simulink model "sensors_actuators"  (Simulink 6.4)
settings: Solver=ode45  StartTime=0.0  StopTime=10.0  RelTol=1e-3
undefined symbols (not defined in the file or in its folder): max_XXX, min_XXX, noiseseed_XXX, noisesource_XXX, std_XXX, T0_XXX, T_XXX, useideal_XXX, usenoise_XXX, XXX
settings Model: Creator=ielulf  LastModifiedBy=ielulf  ExtModeAutoUpdateStatusClock=off

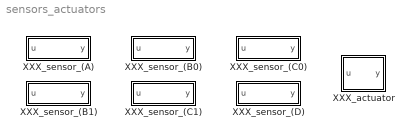
== system sensors_actuators ==
  XXX_actuator : Subsystem
  XXX_sensor_(A) : Subsystem
  XXX_sensor_(B0) : Subsystem
  XXX_sensor_(B1) : Subsystem
  XXX_sensor_(C0) : Subsystem
  XXX_sensor_(C1) : Subsystem
  XXX_sensor_(D) : Subsystem

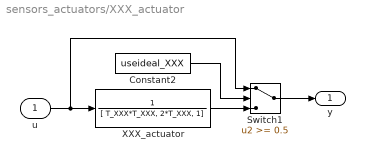
== system sensors_actuators/XXX_actuator ==
  u : Inport
  Constant2 : Constant  Value=useideal_XXX
  Switch1 : Switch  Threshold=0.5
  XXX_actuator : TransferFcn  Denominator=[ T_XXX*T_XXX, 2*T_XXX, 1]
  y : Outport
  wires:
  Constant2/1 -> Switch1/2
  XXX_actuator/1 -> Switch1/3
  Switch1/1 -> y/1
  u/1 -> Switch1/1, XXX_actuator/1

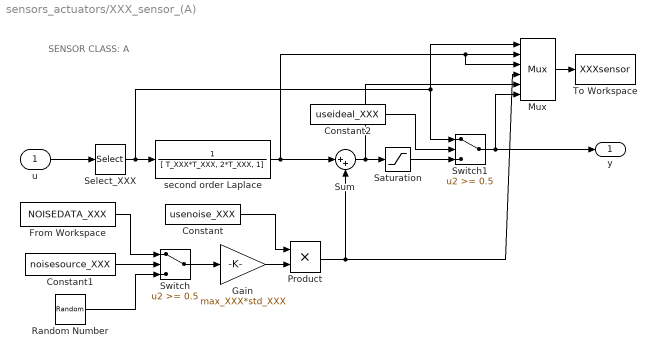
== system sensors_actuators/XXX_sensor_(A) ==
  note: SENSOR CLASS: A
  u : Inport
  Constant : Constant  Value=usenoise_XXX
  Constant1 : Constant  Value=noisesource_XXX
  Constant2 : Constant  Value=useideal_XXX
  From Workspace : FromWorkspace  VariableName=NOISEDATA_XXX  SampleTime=0
  Gain : Gain  Gain=max_XXX*std_XXX  SaturateOnIntegerOverflow=on
  Mux : Mux  Inputs=6
  Product : Product  SaturateOnIntegerOverflow=on  InputSameDT=on
  Random Number : RandomNumber  Seed=noiseseed_XXX  SampleTime=1/1440
  Saturation : Saturate  UpperLimit=max_XXX  LowerLimit=min_XXX
  Select_XXX : Selector  Elements=[XXX]  InputPortWidth=15
  Sum : Sum  Inputs=|++  SaturateOnIntegerOverflow=on  InputSameDT=on
  Switch : Switch  Threshold=0.5
  Switch1 : Switch  Threshold=0.5
  To Workspace : ToWorkspace  VariableName=XXXsensor  SampleTime=-1  SaveFormat=Array
  second order Laplace : TransferFcn  Denominator=[ T_XXX*T_XXX, 2*T_XXX, 1]
  y : Outport
  wires:
  Sum/1 -> Saturation/1, Mux/5
  second order Laplace/1 -> Sum/1, Mux/2, Mux/3
  Product/1 -> Sum/2, Mux/4
  u/1 -> Select_XXX/1
  Select_XXX/1 -> second order Laplace/1, Switch1/1, Mux/1
  Gain/1 -> Product/2
  Switch/1 -> Gain/1
  Constant/1 -> Product/1
  From Workspace/1 -> Switch/1
  Constant1/1 -> Switch/2
  Random Number/1 -> Switch/3
  Saturation/1 -> Switch1/3
  Switch1/1 -> y/1, Mux/6
  Constant2/1 -> Switch1/2
  Mux/1 -> To Workspace/1

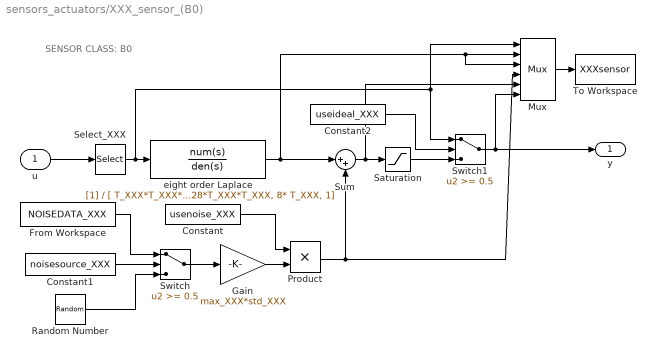
== system sensors_actuators/XXX_sensor_(B0) ==
  note: SENSOR CLASS: B0
  u : Inport
  Constant : Constant  Value=usenoise_XXX
  Constant1 : Constant  Value=noisesource_XXX
  Constant2 : Constant  Value=useideal_XXX
  From Workspace : FromWorkspace  VariableName=NOISEDATA_XXX  SampleTime=0
  Gain : Gain  Gain=max_XXX*std_XXX  SaturateOnIntegerOverflow=on
  Mux : Mux  Inputs=6
  Product : Product  SaturateOnIntegerOverflow=on  InputSameDT=on
  Random Number : RandomNumber  Seed=noiseseed_XXX  SampleTime=1/1440
  Saturation : Saturate  UpperLimit=max_XXX  LowerLimit=min_XXX
  Select_XXX : Selector  Elements=[XXX]  InputPortWidth=15
  Sum : Sum  Inputs=|++  SaturateOnIntegerOverflow=on  InputSameDT=on
  Switch : Switch  Threshold=0.5
  Switch1 : Switch  Threshold=0.5
  To Workspace : ToWorkspace  VariableName=XXXsensor  SampleTime=-1  SaveFormat=Array
  eight order Laplace : TransferFcn  Denominator=[ T_XXX*T_XXX*T_XXX*T_XXX*T_XXX*T_XXX*T_XXX*T_XXX, 8*T_XXX*T_XXX*T_XXX*T_XXX*T_XXX*T_XXX*T_XXX, 28*T_XXX*T_XXX*T_XXX*T_XXX*T_XXX*T_XXX, 56*T_XXX*T_XXX*T_XXX*T_XXX*T_XXX, 70*T_XXX*T_XXX*T_XXX*T_XXX, 56*T_XXX*T_XXX*T_XXX, 28*T_XXX*T_XXX, 8* T_XXX, 1]
  y : Outport
  wires:
  Sum/1 -> Saturation/1, Mux/5
  eight order Laplace/1 -> Sum/1, Mux/2, Mux/3
  Product/1 -> Sum/2, Mux/4
  u/1 -> Select_XXX/1
  Select_XXX/1 -> eight order Laplace/1, Switch1/1, Mux/1
  Gain/1 -> Product/2
  Switch/1 -> Gain/1
  Constant/1 -> Product/1
  From Workspace/1 -> Switch/1
  Constant1/1 -> Switch/2
  Random Number/1 -> Switch/3
  Saturation/1 -> Switch1/3
  Switch1/1 -> y/1, Mux/6
  Constant2/1 -> Switch1/2
  Mux/1 -> To Workspace/1

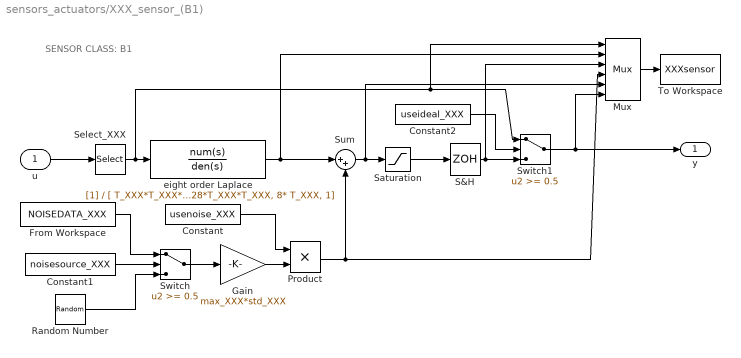
== system sensors_actuators/XXX_sensor_(B1) ==
  note: SENSOR CLASS: B1
  u : Inport
  Constant : Constant  Value=usenoise_XXX
  Constant1 : Constant  Value=noisesource_XXX
  Constant2 : Constant  Value=useideal_XXX
  From Workspace : FromWorkspace  VariableName=NOISEDATA_XXX  SampleTime=0
  Gain : Gain  Gain=max_XXX*std_XXX  SaturateOnIntegerOverflow=on
  Mux : Mux  Inputs=6
  Product : Product  SaturateOnIntegerOverflow=on  InputSameDT=on
  Random Number : RandomNumber  Seed=noiseseed_XXX  SampleTime=1/1440
  S&H : ZeroOrderHold  SampleTime=T0_XXX
  Saturation : Saturate  UpperLimit=max_XXX  LowerLimit=min_XXX
  Select_XXX : Selector  Elements=[XXX]  InputPortWidth=15
  Sum : Sum  Inputs=|++  SaturateOnIntegerOverflow=on  InputSameDT=on
  Switch : Switch  Threshold=0.5
  Switch1 : Switch  Threshold=0.5
  To Workspace : ToWorkspace  VariableName=XXXsensor  SampleTime=-1  SaveFormat=Array
  eight order Laplace : TransferFcn  Denominator=[ T_XXX*T_XXX*T_XXX*T_XXX*T_XXX*T_XXX*T_XXX*T_XXX, 8*T_XXX*T_XXX*T_XXX*T_XXX*T_XXX*T_XXX*T_XXX, 28*T_XXX*T_XXX*T_XXX*T_XXX*T_XXX*T_XXX, 56*T_XXX*T_XXX*T_XXX*T_XXX*T_XXX, 70*T_XXX*T_XXX*T_XXX*T_XXX, 56*T_XXX*T_XXX*T_XXX, 28*T_XXX*T_XXX, 8* T_XXX, 1]
  y : Outport
  wires:
  Switch1/1 -> Mux/6, y/1
  Constant2/1 -> Switch1/2
  S&H/1 -> Mux/3, Switch1/3
  Saturation/1 -> S&H/1
  Sum/1 -> Saturation/1, Mux/5
  eight order Laplace/1 -> Mux/2, Sum/1
  Product/1 -> Sum/2, Mux/4
  u/1 -> Select_XXX/1
  Select_XXX/1 -> Switch1/1, Mux/1, eight order Laplace/1
  Gain/1 -> Product/2
  Switch/1 -> Gain/1
  Constant/1 -> Product/1
  From Workspace/1 -> Switch/1
  Constant1/1 -> Switch/2
  Random Number/1 -> Switch/3
  Mux/1 -> To Workspace/1

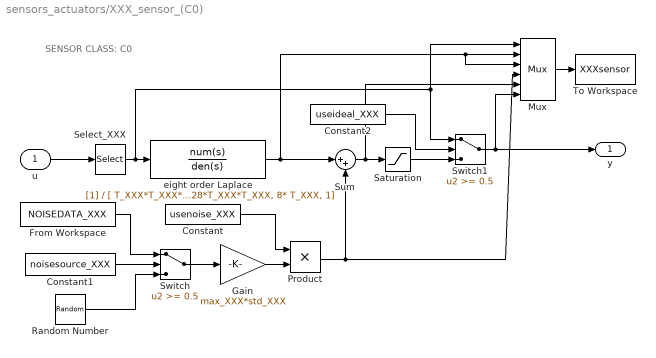
== system sensors_actuators/XXX_sensor_(C0) ==
  note: SENSOR CLASS: C0
  u : Inport
  Constant : Constant  Value=usenoise_XXX
  Constant1 : Constant  Value=noisesource_XXX
  Constant2 : Constant  Value=useideal_XXX
  From Workspace : FromWorkspace  VariableName=NOISEDATA_XXX  SampleTime=0
  Gain : Gain  Gain=max_XXX*std_XXX  SaturateOnIntegerOverflow=on
  Mux : Mux  Inputs=6
  Product : Product  SaturateOnIntegerOverflow=on  InputSameDT=on
  Random Number : RandomNumber  Seed=noiseseed_XXX  SampleTime=1/1440
  Saturation : Saturate  UpperLimit=max_XXX  LowerLimit=min_XXX
  Select_XXX : Selector  Elements=[XXX]  InputPortWidth=15
  Sum : Sum  Inputs=|++  SaturateOnIntegerOverflow=on  InputSameDT=on
  Switch : Switch  Threshold=0.5
  Switch1 : Switch  Threshold=0.5
  To Workspace : ToWorkspace  VariableName=XXXsensor  SampleTime=-1  SaveFormat=Array
  eight order Laplace : TransferFcn  Denominator=[ T_XXX*T_XXX*T_XXX*T_XXX*T_XXX*T_XXX*T_XXX*T_XXX, 8*T_XXX*T_XXX*T_XXX*T_XXX*T_XXX*T_XXX*T_XXX, 28*T_XXX*T_XXX*T_XXX*T_XXX*T_XXX*T_XXX, 56*T_XXX*T_XXX*T_XXX*T_XXX*T_XXX, 70*T_XXX*T_XXX*T_XXX*T_XXX, 56*T_XXX*T_XXX*T_XXX, 28*T_XXX*T_XXX, 8* T_XXX, 1]
  y : Outport
  wires:
  Sum/1 -> Saturation/1, Mux/5
  eight order Laplace/1 -> Sum/1, Mux/2, Mux/3
  Product/1 -> Sum/2, Mux/4
  u/1 -> Select_XXX/1
  Select_XXX/1 -> eight order Laplace/1, Switch1/1, Mux/1
  Gain/1 -> Product/2
  Switch/1 -> Gain/1
  Constant/1 -> Product/1
  From Workspace/1 -> Switch/1
  Constant1/1 -> Switch/2
  Random Number/1 -> Switch/3
  Saturation/1 -> Switch1/3
  Switch1/1 -> y/1, Mux/6
  Constant2/1 -> Switch1/2
  Mux/1 -> To Workspace/1

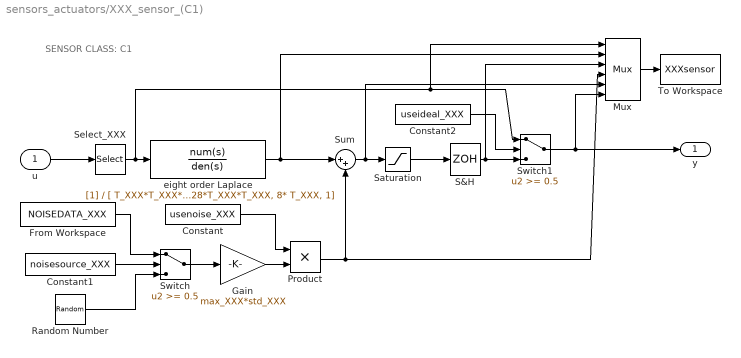
== system sensors_actuators/XXX_sensor_(C1) ==
  note: SENSOR CLASS: C1
  u : Inport
  Constant : Constant  Value=usenoise_XXX
  Constant1 : Constant  Value=noisesource_XXX
  Constant2 : Constant  Value=useideal_XXX
  From Workspace : FromWorkspace  VariableName=NOISEDATA_XXX  SampleTime=0
  Gain : Gain  Gain=max_XXX*std_XXX  SaturateOnIntegerOverflow=on
  Mux : Mux  Inputs=6
  Product : Product  SaturateOnIntegerOverflow=on  InputSameDT=on
  Random Number : RandomNumber  Seed=noiseseed_XXX  SampleTime=1/1440
  S&H : ZeroOrderHold  SampleTime=T0_XXX
  Saturation : Saturate  UpperLimit=max_XXX  LowerLimit=min_XXX
  Select_XXX : Selector  Elements=[XXX]  InputPortWidth=15
  Sum : Sum  Inputs=|++  SaturateOnIntegerOverflow=on  InputSameDT=on
  Switch : Switch  Threshold=0.5
  Switch1 : Switch  Threshold=0.5
  To Workspace : ToWorkspace  VariableName=XXXsensor  SampleTime=-1  SaveFormat=Array
  eight order Laplace : TransferFcn  Denominator=[ T_XXX*T_XXX*T_XXX*T_XXX*T_XXX*T_XXX*T_XXX*T_XXX, 8*T_XXX*T_XXX*T_XXX*T_XXX*T_XXX*T_XXX*T_XXX, 28*T_XXX*T_XXX*T_XXX*T_XXX*T_XXX*T_XXX, 56*T_XXX*T_XXX*T_XXX*T_XXX*T_XXX, 70*T_XXX*T_XXX*T_XXX*T_XXX, 56*T_XXX*T_XXX*T_XXX, 28*T_XXX*T_XXX, 8* T_XXX, 1]
  y : Outport
  wires:
  Switch1/1 -> Mux/6, y/1
  Constant2/1 -> Switch1/2
  S&H/1 -> Mux/3, Switch1/3
  Saturation/1 -> S&H/1
  Sum/1 -> Saturation/1, Mux/5
  eight order Laplace/1 -> Mux/2, Sum/1
  Product/1 -> Sum/2, Mux/4
  u/1 -> Select_XXX/1
  Select_XXX/1 -> Switch1/1, Mux/1, eight order Laplace/1
  Gain/1 -> Product/2
  Switch/1 -> Gain/1
  Constant/1 -> Product/1
  From Workspace/1 -> Switch/1
  Constant1/1 -> Switch/2
  Random Number/1 -> Switch/3
  Mux/1 -> To Workspace/1

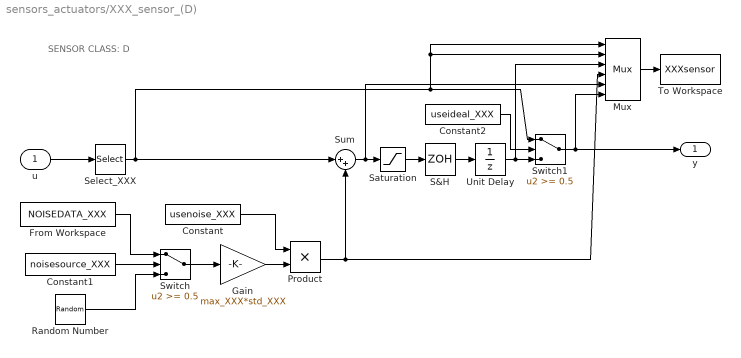
== system sensors_actuators/XXX_sensor_(D) ==
  note: SENSOR CLASS: D
  u : Inport
  Constant : Constant  Value=usenoise_XXX
  Constant1 : Constant  Value=noisesource_XXX
  Constant2 : Constant  Value=useideal_XXX
  From Workspace : FromWorkspace  VariableName=NOISEDATA_XXX  SampleTime=0
  Gain : Gain  Gain=max_XXX*std_XXX  SaturateOnIntegerOverflow=on
  Mux : Mux  Inputs=6
  Product : Product  SaturateOnIntegerOverflow=on  InputSameDT=on
  Random Number : RandomNumber  Seed=noiseseed_XXX  SampleTime=1/1440
  S&H : ZeroOrderHold  SampleTime=T0_XXX
  Saturation : Saturate  UpperLimit=max_XXX  LowerLimit=min_XXX
  Select_XXX : Selector  Elements=[XXX]  InputPortWidth=15
  Sum : Sum  Inputs=|++  SaturateOnIntegerOverflow=on  InputSameDT=on
  Switch : Switch  Threshold=0.5
  Switch1 : Switch  Threshold=0.5
  To Workspace : ToWorkspace  VariableName=XXXsensor  SampleTime=-1  SaveFormat=Array
  Unit Delay : UnitDelay  SampleTime=T0_XXX
  y : Outport
  wires:
  Unit Delay/1 -> Mux/3, Switch1/3
  Constant2/1 -> Switch1/2
  S&H/1 -> Unit Delay/1
  Switch1/1 -> Mux/6, y/1
  Saturation/1 -> S&H/1
  Sum/1 -> Saturation/1, Mux/5
  Product/1 -> Sum/2, Mux/4
  u/1 -> Select_XXX/1
  Select_XXX/1 -> Sum/1, Mux/2, Mux/1, Switch1/1
  Gain/1 -> Product/2
  Switch/1 -> Gain/1
  Constant/1 -> Product/1
  From Workspace/1 -> Switch/1
  Constant1/1 -> Switch/2
  Random Number/1 -> Switch/3
  Mux/1 -> To Workspace/1
